simulink model "model1"  (R2024a)
settings: Solver=ode23t  StartTime=0.0  StopTime=TimeMax  MaxStep=0.1  RelTol=1e-3
model workspace (MAT data in the model file):
  con = [27 27 27 27 27 27 27 28 28 27 27 28 28 28 27 28 28 28 28 28 28 27 28 28 29 27 29 27 27 27 21 21 21 22 21 21 21 22 21 21 21 21 21 21 21 21 22 21 22 22 21 21 21 22 22 22 22 21 22 25]
  liat = [28 27 27 29 29 28 28 28 29 29 28 30 28 27 28 28 27 29 28 28 27 28 29 29 27 27 27 27 27 28 28 29 28 27 29 28 29 28 29 29 28 29 29 29 29 29 28 28 28 27 29 28 29 28 28 29 29 29 27 27 28 28 28 28 27 29 28 28 28 29 29 27 28 29 28 23 23 23 25 24 24 24 24 25 24 24 23 22 23 23 23 23 24 23 23 23 24 24 23 23 23 23 23 23 24 24 24 23 23 24 24 24 24 23 24 24 25 23 24 25 24 24 24 23 23 24 24 23 24 24 24 24 23 22 22 23 24 23 23 23 24 22 23 24 24 23 23 24 23 60]
  novar = 30
  varray = [28 29 27 30 26 28 29 27 25 30 28 29 26 27 28 25 29 30 27 28 27 29 28 30 26 27 29 28 26 27 23 24 22 25 21 23 24 22 20 25 23 24 21 22 23 20 24 25 22 21 23 24 22 25 21 22 24 25 22 15]
values from neighbouring files (symbols this model uses):
  AirDensity = 1.225    [model_variables.mat]    (also in var.m)
  AttemptData = readtable('TrackModel\410-3.csv')    [var.m]
  CD = 0.1495849    [model_variables.mat]    (also in var.m)
  CRR = 0.0015    [model_variables.mat]    (also in var.m)
  DistancetoGlide = 13301    [model_variables.mat]    (also in var.m)
  FrontArea = 0.42941    [model_variables.mat]    (also in var.m)
  FrontAxle = 510.7    [model_variables.mat]    (also in var.m)
  FrontGear = 11    [model_variables.mat]    (also in var.m)
  Gravitation = 9.80665    [model_variables.mat]    (also in var.m)
  MassWheel = 1    [model_variables.mat]    (also in var.m)
  NewData = TrackData(:, {'s', 'gradient_rad'})    [var.m]
  RadiusWheel = 0.25    [model_variables.mat]    (also in var.m)
  RearAxle = 1504.27    [model_variables.mat]    (also in var.m)
  RearGear = 142    [model_variables.mat]    (also in var.m)
  SlipAngle = 0.03    [model_variables.mat]    (also in var.m)
  SpeedData = readtable('TrackModel\KMHE3Speed.csv')    [var.m]
  TrackData = readtable('Track\Path\ePrix\mincurvfinal_ePrix_nonsmoothedgrad.csv')    [var.m]
  VehicleMass = 76    [model_variables.mat]    (also in var.m)
undefined symbols (not defined in the file or in its folder): finalatt, StateData
libraries: fl_lib x18, nesl_utility x15, sdl_lib x7, ee_lib x2, batteryecm_lib x1
(part 1 of 2)
settings Model: Creator=baiqu  LastModifiedBy=baiqu
settings SolverCC: MaxConsecutiveMinStep=5  ZeroCrossAlgorithm=Adaptive  AlgebraicLoopSolver=TrustRegion
settings DataIOCC: ReturnWorkspaceOutputs=off
settings DebuggingCC: IgnoredZcDiagnostic=none

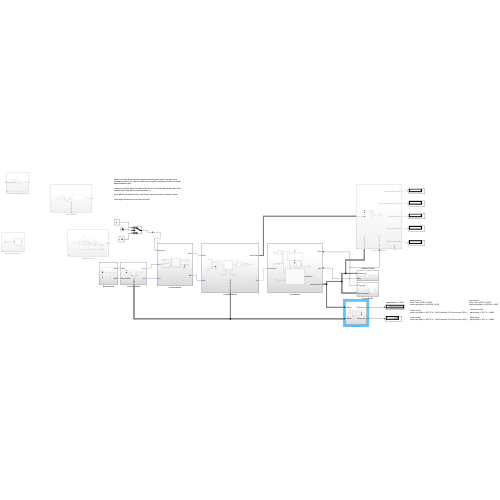
[thumbnail: Simulink's stored preview of the top-level diagram]
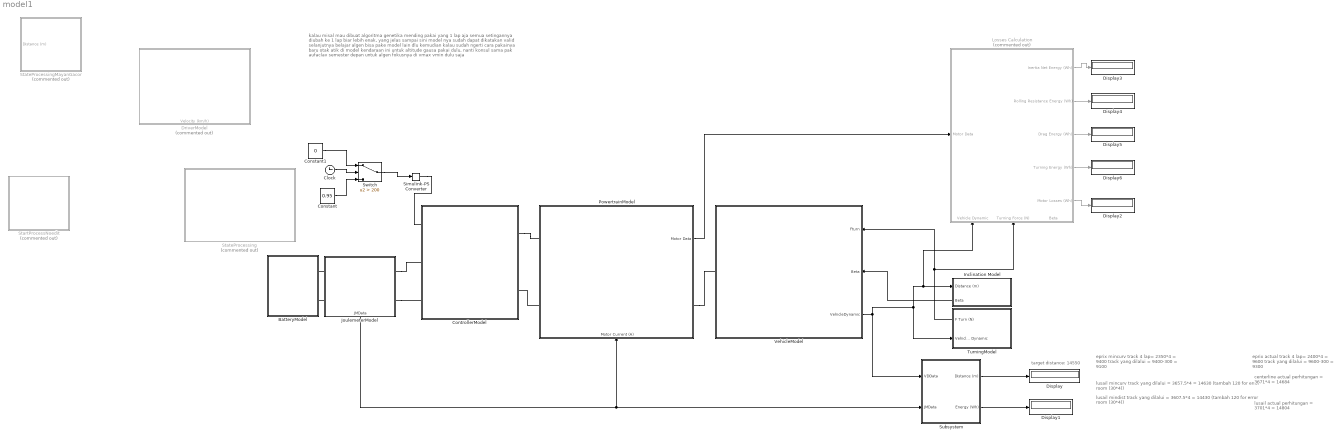
== system model1 ==
  note: target distance: 14550
  note: kalau misal mau dibuat algoritma genetika mending pakai yang 1 lap aja semua setingannya diubah ke 1 lap biar lebih enak, yang jelas sampai sini model nya sudah dapat dikatakan valid
      |
      | selanjutnya belajar algen bisa pake model lain dlu kemudian kalau sudah ngerti cara pakainya baru otak atik di model kendaraan ini
      |
      | untuk altitude gausa pakai dulu, nanti konsul sama pak aufaclav semester depan
      |
      | untuk algen fokusnya di vmax vmin dulu saja
  note: eprix actual
      | track 4 lap= 2400*4 = 9600
      | track yang dilalui = 9600-300 = 9300
  note: lusail actual
      | perhitungan = 3701*4 = 14804
  note: eprix mincurv
      | track 4 lap= 2350*4 = 9400
      | track yang dilalui = 9400-300 = 9100
  note: lusail mindist
      | track yang dilalui = 3607.5*4 = 14430 (tambah 120 for error room (30*4))
  note: lusail mincurv
      | track yang dilalui = 3657.5*4 = 14630 (tambah 120 for error room (30*4))
  note: centerline actual
      | perhitungan = 3671*4 = 14684
  BatteryModel : Subsystem
  Clock : Clock
  Constant : Constant  Value=0.95
  Constant1 : Constant  Value=0
  ControllerModel : Subsystem
  Display{,1..6} (7 alike) : Display
  DriverModel : Subsystem  Commented=on
      settings: PortSchema="{\"entries\":[{\"content\":{\"sides\":[{\"content\":{},\"type\":\"ConnectorPlacement.EquallySpacedRectSide\",\"uuid\":\"89714f29-06d9-46e2-b121-09eafd11e56c\"},{\"content\":{\"connectorIds\":[\"RConn1\"],\"side\":\"RIGHT\"},\"type\":\"ConnectorPlacement.EquallySpacedRectSide\",\"uuid\":\"45c8a396-5542-43c7-a708-f386e71eba33\"},{\"content\":{\"side\":\"TOP\"},\"type\":\"ConnectorPlacement.EquallySpacedRectSide\",\"uuid\":\"8953ccf4-c3cd-467e-b5a0-b03c7ca56c90\"},{\"content\":{\"connectorIds\":[\"In1\"],\"side\":\"BOTTOM\"},\"type\":\"ConnectorPlacement.EquallySpacedRectSide\",\"uuid\":\"ab8b1a80-a65e-491d-931c-f50f5886be3d\"}]},\"type\":\"ConnectorPlacement.EquallySpacedConnector\",\"uuid\":\"4bd302de-f506-487a-9315-f217838135a7\"}],\"packageUris\":[\"http://schema.mathworks.com/mf0/Connector/R2020b\"],\"version\":\"1.0\"}"
  Inclination Model : Subsystem
      settings: PortSchema="{\"entries\":[{\"content\":{\"sides\":[{\"content\":{},\"type\":\"ConnectorPlacement.EquallySpacedRectSide\",\"uuid\":\"136e15b9-992d-4bd3-9ecd-22bc584851ec\"},{\"content\":{\"connectorIds\":[\"In1\",\"Out1\"],\"side\":\"RIGHT\"},\"type\":\"ConnectorPlacement.EquallySpacedRectSide\",\"uuid\":\"21901198-73a1-4f2b-bd2a-55a4ec918fc9\"},{\"content\":{\"side\":\"TOP\"},\"type\":\"ConnectorPlacement.EquallySpacedRectSide\",\"uuid\":\"96b62914-b1ee-40c2-9187-7fe30b0e8d87\"}]},\"type\":\"ConnectorPlacement.EquallySpacedConnector\",\"uuid\":\"3de7d7f5-6cf3-49e2-811a-f65baadaba13\"}],\"packageUris\":[\"http://schema.mathworks.com/mf0/Connector/R2020b\"],\"version\":\"1.0\"}"
  JoulemeterModel : Subsystem
      settings: PortSchema="{\"entries\":[{\"content\":{\"sides\":[{\"content\":{\"connectorIds\":[\"LConn1\",\"LConn2\"]},\"type\":\"ConnectorPlacement.EquallySpacedRectSide\",\"uuid\":\"5b7f183a-bf7a-4999-b582-2617b2cbf3b5\"},{\"content\":{\"connectorIds\":[\"RConn1\",\"RConn2\"],\"side\":\"RIGHT\"},\"type\":\"ConnectorPlacement.EquallySpacedRectSide\",\"uuid\":\"60e6a297-a548-4f80-bd0a-fa1cc363ffaf\"},{\"content\":{\"side\":\"TOP\"},\"type\":\"ConnectorPlacement.EquallySpacedRectSide\",\"uuid\":\"7f0257a8-d3f8-4392-a80f-b293aa05a497\"},{\"content\":{\"connectorIds\":[\"Out1\"],\"side\":\"BOTTOM\"},\"type\":\"ConnectorPlacement.EquallySpacedRectSide\",\"uuid\":\"bc8eaeec-fb49-4b5e-9f30-46577002e429\"}]},\"type\":\"ConnectorPlacement.EquallySpacedConnector\",\"uuid\":\"4d471f89-f217-48cc-a8db-ea855d9b8dd6\"}],\"packageUris\":[\"http://schema.mathworks.com/mf0/Connector/R2020b\"],\"version\":\"1.0\"}"
  Losses Calculation : Subsystem  Commented=on
      settings: PortSchema="{\"entries\":[{\"content\":{\"sides\":[{\"content\":{\"connectorIds\":[\"In1\"]},\"type\":\"ConnectorPlacement.EquallySpacedRectSide\",\"uuid\":\"1b3e4d1e-49e6-427b-8c70-72d72d3276fb\"},{\"content\":{\"connectorIds\":[\"Out1\",\"Out2\",\"Out3\",\"Out4\",\"Out5\"],\"side\":\"RIGHT\"},\"type\":\"ConnectorPlacement.EquallySpacedRectSide\",\"uuid\":\"db691218-5a1c-4b6a-822c-f6125d5f80f1\"},{\"content\":{\"side\":\"TOP\"},\"type\":\"ConnectorPlacement.EquallySpacedRectSide\",\"uuid\":\"d328adc1-9cf5-4bdc-bff5-091ed8789e88\"},{\"content\":{\"connectorIds\":[\"In2\",\"In3\",\"In4\"],\"side\":\"BOTTOM\"},\"type\":\"ConnectorPlacement.EquallySpacedRectSide\",\"uuid\":\"bf96b796-aa10-4143-8481-077c36306021\"}]},\"type\":\"ConnectorPlacement.EquallySpacedConnector\",\"uuid\":\"61290827-2b1b-4af0-b2c2-32cdcb45fb74\"}],\"packageUris\":[\"http://schema.mathworks.com/mf0/Connector/R2020b\"],\"version\":\"1.0\"}"
  PowertrainModel : Subsystem
      settings: PortSchema="{\"entries\":[{\"content\":{\"sides\":[{\"content\":{\"connectorIds\":[\"LConn1\",\"LConn2\"]},\"type\":\"ConnectorPlacement.EquallySpacedRectSide\",\"uuid\":\"d69fc031-75de-46f6-9385-72f54b88d1cb\"},{\"content\":{\"connectorIds\":[\"Out1\",\"RConn1\"],\"side\":\"RIGHT\"},\"type\":\"ConnectorPlacement.EquallySpacedRectSide\",\"uuid\":\"3d253726-be1e-4202-97ec-580b8e540a5a\"},{\"content\":{\"side\":\"TOP\"},\"type\":\"ConnectorPlacement.EquallySpacedRectSide\",\"uuid\":\"cefbe44c-5e87-4e34-a220-1e2cd8a2aa2e\"},{\"content\":{\"connectorIds\":[\"In1\"],\"side\":\"BOTTOM\"},\"type\":\"ConnectorPlacement.EquallySpacedRectSide\",\"uuid\":\"e2aebd15-c630-4215-8d14-672c4b032223\"}]},\"type\":\"ConnectorPlacement.EquallySpacedConnector\",\"uuid\":\"d11a7537-5ed0-42cc-8f47-41e0a2228910\"}],\"packageUris\":[\"http://schema.mathworks.com/mf0/Connector/R2020b\"],\"version\":\"1.0\"}"
  Simulink-PS Converter : nesl_utility/Simulink-PS Converter  PhysicalDomain=network_engine_domain  SubClassName=ps_input  LeftPortType=input  RightPortType=output  PseudoPeriodic=off  Frequencies=[]  NoiseDistribution=none  NoiseParameters=[]  Unit=1  AffineConversion=off  FilteringAndDerivatives=provide  SimscapeFilterOrder=1  InputFilterTimeConstant=0.001  UdotUserProvided=0
  StartProcessNoedit : Subsystem  Commented=on
  StateProcessing : Subsystem  Commented=on
  StateProcessingMayanGacor : Subsystem  Commented=on
  Subsystem : Subsystem
  Switch : Switch  Criteria=u2 > Threshold  Threshold=200  SaturateOnIntegerOverflow=off  InputSameDT=off
  TurningModel : Subsystem
      settings: PortSchema="{\"entries\":[{\"content\":{\"sides\":[{\"content\":{\"connectorIds\":[\"Out1\",\"In1\"]},\"type\":\"ConnectorPlacement.EquallySpacedRectSide\",\"uuid\":\"d4692372-87e9-4ce8-a189-eb5e05ef7ce2\"},{\"content\":{\"side\":\"RIGHT\"},\"type\":\"ConnectorPlacement.EquallySpacedRectSide\",\"uuid\":\"c6a7fc47-7281-4ca2-ad0e-ceadd6b2be83\"},{\"content\":{\"side\":\"TOP\"},\"type\":\"ConnectorPlacement.EquallySpacedRectSide\",\"uuid\":\"b8ded78c-a4e7-43a6-a6ec-269e22706b6e\"}]},\"type\":\"ConnectorPlacement.EquallySpacedConnector\",\"uuid\":\"a77bfcc2-1edf-497f-8c86-74b621a681e7\"}],\"packageUris\":[\"http://schema.mathworks.com/mf0/Connector/R2020b\"],\"version\":\"1.0\"}"
  VehicleModel : Subsystem
      settings: PortSchema="{\"entries\":[{\"content\":{\"sides\":[{\"content\":{\"connectorIds\":[\"LConn1\"]},\"type\":\"ConnectorPlacement.EquallySpacedRectSide\",\"uuid\":\"93bb66e9-fe50-4a31-bb73-2398351c668b\"},{\"content\":{\"connectorIds\":[\"In1\",\"In2\",\"Out1\"],\"side\":\"RIGHT\"},\"type\":\"ConnectorPlacement.EquallySpacedRectSide\",\"uuid\":\"0cd3e741-0813-4587-beb9-127565be059b\"},{\"content\":{\"side\":\"TOP\"},\"type\":\"ConnectorPlacement.EquallySpacedRectSide\",\"uuid\":\"8c668a08-9049-4798-9275-4c55ebdb510f\"}]},\"type\":\"ConnectorPlacement.EquallySpacedConnector\",\"uuid\":\"e7ef1dcb-e51f-4722-9d73-8e83c911e490\"}],\"packageUris\":[\"http://schema.mathworks.com/mf0/Connector/R2020b\"],\"version\":\"1.0\"}"
  wires:
  JoulemeterModel/1(JMData) -> PowertrainModel/1(Motor Current (A)), Subsystem/2(JMData)
  TurningModel/1(F Turn (N)) -> VehicleModel/1(Fturn), Losses Calculation/3(Turning Force (N))
  Subsystem/1(Distance (m)) -> Display/1
  Subsystem/2(Energy (Wh)) -> Display1/1
  VehicleModel/1(VehicleDynamic) -> Losses Calculation/2(Vehicle Dynamic), Inclination Model/1(Distance (m)), TurningModel/1(Vehicle Dynamic), Subsystem/1(VDData)
  PowertrainModel/1(Motor Data) -> Losses Calculation/1(Motor Data)
  Losses Calculation/4(Turning Energy (Wh)) -> Display6/1
  Losses Calculation/3(Drag Energy (Wh)) -> Display5/1
  Losses Calculation/2(Rolling Resistance Energy (Wh)) -> Display4/1
  Losses Calculation/1(Inertia Net Energy (Wh)) -> Display3/1
  Inclination Model/1(Beta) -> VehicleModel/2(Beta)
  Losses Calculation/5(Motor Losses (Wh)) -> Display2/1
  Switch/1 -> Simulink-PS Converter/1
  Clock/1 -> Switch/2
  Constant1/1 -> Switch/1
  Constant/1 -> Switch/3
  connections:
  PowertrainModel/LConn2 -- ControllerModel/RConn2
  ControllerModel/RConn1 -- PowertrainModel/LConn1
  PowertrainModel/RConn1 -- VehicleModel/LConn1
  JoulemeterModel/RConn1 -- ControllerModel/LConn2
  JoulemeterModel/RConn2 -- ControllerModel/LConn3
  JoulemeterModel/LConn1 -- BatteryModel/RConn1
  JoulemeterModel/LConn2 -- BatteryModel/RConn2
  Simulink-PS Converter/RConn1 -- ControllerModel/LConn1

== system model1/BatteryModel ==
  Battery : batteryecm_lib/Battery  Vnom=Vnom V  prm_dir=simscape.enum.battery.prm_dir.disabled  R1_dis=2 Ohm  R1_ch=2 Ohm  R1=RintBat mOhm  prm_AH=simscape.enum.battery.prm_AH.infinite  AH=50 A*hr  V1=11.5 V  AH1=25 A*hr  prm_R2=simscape.enum.battery.prm_R2.disabled  R2=2000 Ohm  Tmeas=298.15 K  charge_measurement_port=simscape.enum.battery.enable.no  prm_dyn=simscape.enum.battery.prm_dyn.off  Rp1=0.005 Ohm  tau1=30 s  Rp2=0.005 Ohm  tau2=30 s  Rp3=0.005 Ohm  tau3=30 s  Rp4=0.005 Ohm  tau4=30 s  Rp5=0.005 Ohm  tau5=30 s  prm_fade=simscape.enum.battery.prm_fade.disabled  N_fade=100  AH_fade=45 A*hr  R1_fade=2.02 Ohm  R1_ch_fade=2.02 Ohm  V1_fade=10.35 V  prm_age=simscape.enum.battery.prm_age.disabled  prm_age_OCV=simscape.enum.battery.prm_age_OCV.OCV  OCV_age=0.9  SOC_age=60  Tmeas_age=298.15 K  delta_time_age_vec=[0] d  temperature_age_vec=[273] K  OCV_scaling_age=2.2134e6  OCV_offset_age=1.632e6  temp_exp_age=0.515833569 V  t_exp_age=0.75  Vnom_T2=12 V  R1_T2=2.2 Ohm  R1_T2_dis=2.2 Ohm  R1_T2_ch=2.2 Ohm  V1_T2=11.4 V  R2_T2=2200 Ohm  Rp1_T2=0.005 Ohm  tau1_T2=30 s  Rp2_T2=0.005 Ohm  tau2_T2=30 s  Rp3_T2=0.005 Ohm  tau3_T2=30 s  Rp4_T2=0.005 Ohm  tau4_T2=30 s  Rp5_T2=0.005 Ohm  tau5_T2=30 s  Tmeas2=273.15 K  thermal_port=simscape.enum.thermaleffects.omit  thermal_mass=30000 J/K  i_specify=off  i_priority=None  i=0 A  i_nominal_specify=off  i_nominal_value=1  i_nominal_unit=A  v_specify=off  v_priority=None  v=0 V  v_nominal_specify=off  v_nominal_value=1  v_nominal_unit=V  charge_specify=off  charge_priority=High  charge=50 A*hr  charge_nominal_specify=off  charge_nominal_value=1  charge_nominal_unit=A*hr  num_cycles_specify=off  num_cycles_priority=High  num_cycles=0  num_cycles_nominal_specify=off  num_cycles_nominal_value=1  num_cycles_nominal_unit=1  temperature_specify=off  temperature_priority=High  temperature=298.15 K  temperature_nominal_specify=off  temperature_nominal_value=1  temperature_nominal_unit=K
  Electrical Reference : fl_lib/Electrical/Electrical Elements/Electrical Reference
  Solver Configuration : nesl_utility/Solver Configuration  PhysicalDomain=network_engine_domain  SubClassName=solver  LeftPortType=input  RightPortType=generic  Tones=[]  Harmonics=[]  SimulateNoise=off  Profile=off  UseLocalSampling=off  EnableSwitchedLinearOptims=on  FrequencyDomain=off  UseCCode=off  RelTol=0.001  AbsTol=0.001  MinStep=1e-09  ToWorkspace=off  RevertToSquareIcSolve=off  NumHomotopyIterations=100  PhasorMode=off  PhasorModeNumHarmonics=1  ConsistencySolver=NEWTON_XTOL_AFTER_FTOL  IndexReductionMethod=DerivativeReplacement  DoDC=off  ResidualTolerance=1e-09  ConsistencyTolSource=GLOBAL  ConsistencyAbsTol=0.001  ConsistencyRelTol=0.001  ConsistencyTolFactor=0.001  UseLocalSolver=off  LocalSolverChoice=NE_BACKWARD_EULER_ADVANCER  ResolveIndetEquations=on  FunctionEvalNumThread=1  LocalSolverSampleTime=0.001  DoFixedCost=off  MaxNonlinIter=3  MaxModeIter=2  ComputeImpulses=off  ImpulseIterations=2  LinearAlgebra=auto  LinearAlgebraNumThread=0  EquationFormulation=NE_TIME_EF  DelaysMemoryBudget=1024  AutomaticFiltering=on  FilteringTimeConstant=0.001  PartitionStorageMethod=AS_NEEDED  PartitionMemoryBudget=1024  PartitionMethod=ROBUST  MultibodyUseLocalSolver=off  MultibodyLocalSolverChoice=ODE1  MultibodyLocalSolverSampleTime=0.001
  Vbus : PMIOPort  Side=Right
  GND : PMIOPort  Port=2  Side=Right
  connections:
  Battery/RConn1 -- GND/RConn1 -- Solver Configuration/RConn1 -- Electrical Reference/LConn1
  Vbus/RConn1 -- Battery/LConn1

== system model1/ControllerModel ==
  Average-Value DC-DC Converter : ee_lib/Semiconductors & Converters/Converters/Average-Value DC-DC Converter  control_option=ee.enum.converters.controlinput.dutycycle  converter_type=ee.enum.converters.dcdctype.buck  efficiency_option=ee.enum.converters.efficiency.constant  efficiency_fixed=100  i_vec=[0, 2, 5] A  efficiency_vec=[90, 95, 98]
      settings: InternalSimscapePortConfiguration="{\"Bottom\":[],\"Left\":[{\"id\":\"DutyCycle\",\"label\":\"DutyCycle\",\"type\":\"input\"},{\"id\":\"p1\",\"label\":\"1+\",\"type\":\"foundation.electrical.electrical\"},{\"id\":\"n1\",\"label\":\"1-\",\"type\":\"foundation.electrical.electrical\"}],\"Right\":[{\"id\":\"p2\",\"label\":\"2+\",\"type\":\"foundation.electrical.electrical\"},{\"id\":\"n2\",\"label\":\"2-\",\"type\":\"foundation.electrical.electrical\"}],\"Top\":[]}"
  Electrical Reference : fl_lib/Electrical/Electrical Elements/Electrical Reference
  DutyCycle : PMIOPort  Side=Left
  Con+ : PMIOPort  Port=2  Side=Left
  Con- : PMIOPort  Port=3  Side=Left
  Mot+ : PMIOPort  Port=4  Side=Right
  Mot- : PMIOPort  Port=5  Side=Right
  connections:
  Average-Value DC-DC Converter/RConn1 -- Mot+/RConn1
  Average-Value DC-DC Converter/LConn1 -- DutyCycle/RConn1
  Average-Value DC-DC Converter/LConn2 -- Con+/RConn1
  Average-Value DC-DC Converter/RConn2 -- Electrical Reference/LConn1 -- Mot-/RConn1
  Average-Value DC-DC Converter/LConn3 -- Con-/RConn1

== system model1/DriverModel ==
  Velocity (km/h) : Inport
  Bus Selector : BusSelector  OutputSignals=Velocity (km/h)
  Constant : Constant  Value=[29 29 28 29 28 28 28 29 29 28 29 28 28 29 28 28 29 27 28 28 28 28 28 28 28 28 28 28 28 28 28 28 29 28 29 28 27 28 29 27 28 28 28 28 28 28 28 29 28 29 28 28 29 29 29 29 27 29 28 28 28 28 28 29 29 28 28 28 29 29 24 23 23 23 23 23 24 25 24 23 23 23 23 23 24 23 23 23 23 23 24 24 24 24 24 24 24 23 24 23 23 24 24 24 24 23 23 23 23 23 23 23 24 24 23 23 23 24 24 23 24 24 25 24 24 22 23 23 23 23 23 23 23 23 24 24 23 24 24 56]
  Constant1 : Constant  Value=70
  MATLAB Function : MATLAB Function  TreatAsAtomicUnit=on
  Memory : Memory
  Memory1 : Memory
  Subsystem : Subsystem
  Transfer Fcn : TransferFcn  Denominator=[1e-10 1]
  DC : PMIOPort  Side=Right
  wires:
  Velocity (km/h)/1 -> Bus Selector/1
  MATLAB Function/1(control) -> Subsystem/1(state)
  MATLAB Function/3(n) -> Memory/1
  Memory1/1 -> MATLAB Function/4(state_prev)
  Memory/1 -> MATLAB Function/5(n_prev)
  Constant1/1 -> MATLAB Function/1(no_var)
  Constant/1 -> MATLAB Function/2(v_array)
  MATLAB Function/2(state) -> Memory1/1
  Bus Selector/1 -> Transfer Fcn/1  "<Velocity (km/h)>"
  Transfer Fcn/1 -> MATLAB Function/3(v)
  connections:
  DC/RConn1 -- Subsystem/RConn1

== system model1/Inclination Model ==
  note: pakai 20
  Distance (m) : Inport
  1-D Lookup Table1 : Lookup_n-D  NumberOfTableDimensions=1  BreakpointsForDimension1=NewData{:,1}  Table=NewData{:,2}  InternalRulePriority=Speed  RndMeth=Simplest
  Bus Selector : BusSelector  OutputSignals=Distance (m),Velocity (km/h)
  Constant : Constant  Value=NewData{end,1}
  Gain : Gain  Gain=1/100
  MATLAB Function1 : MATLAB Function  TreatAsAtomicUnit=on
  Unit Delay : UnitDelay  SampleTime=-1  HasFrameUpgradeWarning=on
  Beta : Outport
  wires:
  MATLAB Function1/1(position) -> 1-D Lookup Table1/1
  Constant/1 -> MATLAB Function1/2(s_track)
  Distance (m)/1 -> Bus Selector/1
  Bus Selector/1 -> Unit Delay/1  "<Distance (m)>"
  1-D Lookup Table1/1 -> Gain/1
  Gain/1 -> Beta/1
  Unit Delay/1 -> MATLAB Function1/1(s)

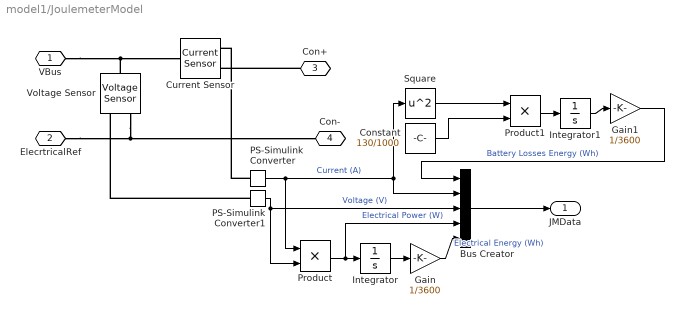
== system model1/JoulemeterModel ==
  Bus Creator : BusCreator  Inputs=5
  Constant : Constant  Value=130/1000
  Current Sensor : fl_lib/Electrical/Electrical Sensors/Current Sensor
  Gain : Gain  Gain=1/3600
  Gain1 : Gain  Gain=1/3600
  Integrator : Integrator
  Integrator1 : Integrator
  PS-Simulink Converter : nesl_utility/PS-Simulink Converter  PhysicalDomain=network_engine_domain  SubClassName=ps_output  LeftPortType=input  RightPortType=output  PseudoPeriodic=off  Frequencies=[]  VectorFormat=1-D array  Unit=A  AffineConversion=off
  PS-Simulink Converter1 : nesl_utility/PS-Simulink Converter  PhysicalDomain=network_engine_domain  SubClassName=ps_output  LeftPortType=input  RightPortType=output  PseudoPeriodic=off  Frequencies=[]  VectorFormat=1-D array  Unit=V  AffineConversion=off
  Product : Product
  Product1 : Product
  Square : Math  Operator=square
  Voltage Sensor : fl_lib/Electrical/Electrical Sensors/Voltage Sensor
  VBus : PMIOPort  Side=Left
  ElecrtricalRef : PMIOPort  Port=2  Side=Left
  Con+ : PMIOPort  Port=3  Side=Right
  Con- : PMIOPort  Port=4  Side=Right
  JMData : Outport
  wires:
  PS-Simulink Converter/1 -> Product/1, Square/1, Bus Creator/2  "Current (A)"
  PS-Simulink Converter1/1 -> Product/2, Bus Creator/3  "Voltage (V)"
  Bus Creator/1 -> JMData/1
  Product/1 -> Integrator/1, Bus Creator/4  "Electrical Power (W)"
  Gain/1 -> Bus Creator/5  "Electrical Energy (Wh)"
  Integrator/1 -> Gain/1
  Constant/1 -> Product1/2
  Square/1 -> Product1/1
  Gain1/1 -> Bus Creator/1  "Battery Losses Energy (Wh)"
  Integrator1/1 -> Gain1/1
  Product1/1 -> Integrator1/1
  connections:
  Voltage Sensor/LConn1 -- VBus/RConn1 -- Current Sensor/LConn1
  Voltage Sensor/RConn2 -- ElecrtricalRef/RConn1 -- Con-/RConn1
  PS-Simulink Converter1/LConn1 -- Voltage Sensor/RConn1
  PS-Simulink Converter/LConn1 -- Current Sensor/RConn1
  Con+/RConn1 -- Current Sensor/RConn2

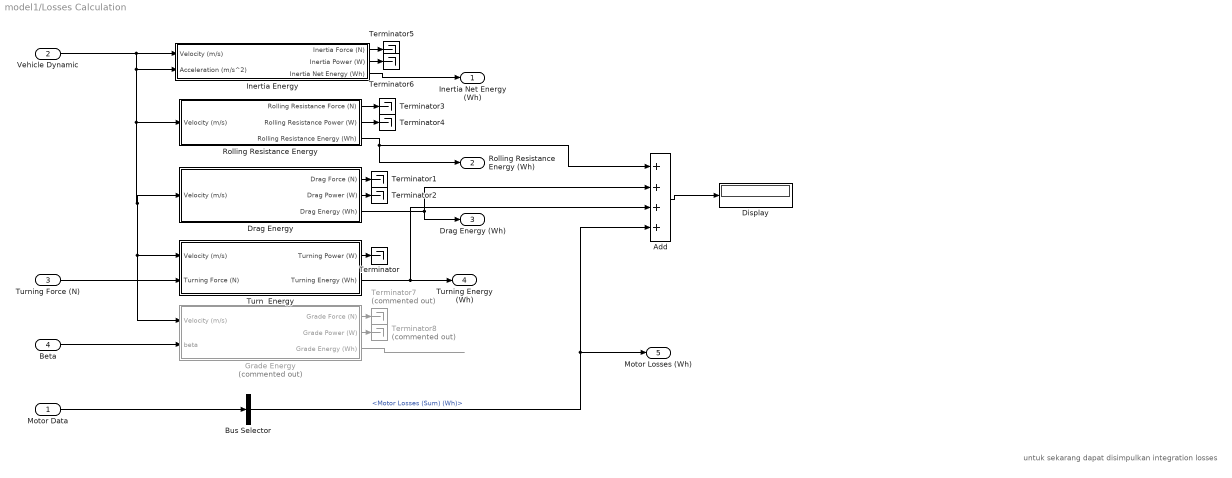
== system model1/Losses Calculation ==
  note: untuk sekarang dapat disimpulkan integration losses
  Motor Data : Inport
  Vehicle Dynamic : Inport  Port=2
  Turning Force (N) : Inport  Port=3
  Beta : Inport  Port=4
  Add : Sum  Inputs=++++
  Bus Selector : BusSelector  OutputSignals=Motor Losses (Sum) (Wh)
  Display : Display
  Drag Energy : Subsystem
  Grade Energy : Subsystem  Commented=on
  Inertia Energy : Subsystem
  Rolling Resistance Energy : Subsystem
  Terminator{,1..6} (7 alike) : Terminator
  Terminator7 : Terminator  Commented=on
  Terminator8 : Terminator  Commented=on
  Turn  Energy : Subsystem
  Inertia Net Energy (Wh) : Outport
  Rolling Resistance Energy (Wh) : Outport  Port=2
  Drag Energy (Wh) : Outport  Port=3
  Turning Energy (Wh) : Outport  Port=4
  Motor Losses (Wh) : Outport  Port=5
  wires:
  Drag Energy/2(Drag Power (W)) -> Terminator2/1
  Inertia Energy/2(Inertia Power (W)) -> Terminator6/1
  Turn  Energy/1(Turning Power (W)) -> Terminator/1
  Inertia Energy/3(Inertia Net Energy (Wh)) -> Inertia Net Energy (Wh)/1
  Drag Energy/1(Drag Force (N)) -> Terminator1/1
  Rolling Resistance Energy/3(Rolling Resistance Energy (Wh)) -> Rolling Resistance Energy (Wh)/1, Add/1
  Vehicle Dynamic/1 -> Grade Energy/1(Velocity (m/s)), Turn  Energy/1(Velocity (m/s)), Drag Energy/1(Velocity (m/s)), Rolling Resistance Energy/1(Velocity (m/s)), Inertia Energy/2(Acceleration (m/s^2)), Inertia Energy/1(Velocity (m/s))
  Rolling Resistance Energy/1(Rolling Resistance Force (N)) -> Terminator3/1
  Inertia Energy/1(Inertia Force (N)) -> Terminator5/1
  Rolling Resistance Energy/2(Rolling Resistance Power (W)) -> Terminator4/1
  Drag Energy/3(Drag Energy (Wh)) -> Drag Energy (Wh)/1, Add/2
  Turn  Energy/2(Turning Energy (Wh)) -> Add/3, Turning Energy (Wh)/1
  Add/1 -> Display/1
  Motor Data/1 -> Bus Selector/1
  Bus Selector/1 -> Add/4, Motor Losses (Wh)/1  "<Motor Losses (Sum) (Wh)>"
  Turning Force (N)/1 -> Turn  Energy/2(Turning Force (N))
  Beta/1 -> Grade Energy/2(beta)
  Grade Energy/3(Grade Energy (Wh)) -> ?
  Grade Energy/1(Grade Force (N)) -> Terminator7/1
  Grade Energy/2(Grade Power (W)) -> Terminator8/1

== system model1/PowertrainModel ==
  Motor Current (A) : Inport
  DC Motor : ee_lib/Electromechanical/Brushed Motors/DC Motor  Tag={'toolbox/physmod/elec/library/m/ee_lib_parts';'Electromechanical/Brushed_Motors/DC_Motor/Maxon/RE_65_388987_48.xml'}  field_option=ee.enum.field_option.pm  Rf=100 % Parameter not set Ohm  Lf=1 % Parameter not set H  Laf=0.15 % Parameter not set H  If0=0 % Parameter not set A  parameterization=ee.enum.dcparam_option.circuit_param  Ra=0.365 Ohm  La=0.161 mH  emf_or_torque=ee.enum.emf_or_torque.ki  Kv=12.88053 % Parameter estimated mV/rpm  Ki=123 mN*m/A  T_stall=0.24e-3 % Parameter not set N*m  w_max=19100 % Parameter not set rpm  w_rated=15000 % Parameter not set rpm  P_rated=0.08 % Parameter not set W  V_rated=1.5 % Parameter not set V  lam_param=ee.enum.lam_param.current  i_noload=0.289 A  V_i_noload=48 V  J=1340 g*cm^2  lam=0 % % Parameter not set mN*m/(rad/s)  speed0=0 % Parameter not set rpm  enable_fault_armature=simscape.enum.onoff.off  rev_faulted=1 / 3 % Parameter not set  G_faulted_armature=1e-5 % Parameter not set S  fault_trigger_armature=ee.enum.faults.faultTrigger.temporal  t_fault_armature=1 % Parameter not set s  max_permissible_current_armature=inf % Parameter not set A  t_fail_on_current_armature=1 % Parameter not set s  enable_fault_field=simscape.enum.onoff.off  G_faulted_field=1e-5 % Parameter not set S  fault_trigger_field=ee.enum.faults.faultTrigger.temporal  t_fault_field=1 % Parameter not set s  max_permissible_current_field=inf % Parameter not set A  t_fail_on_current_field=1 % Parameter not set s  fault_action=simscape.enum.assert.action.none  alpha=3.93e-3 % Parameter not set 1/K  Tmeas=25 % Parameter not set degC  thermal_mass=667.588357588358 % Parameter estimated J/K  initial_temperature=25 % Parameter not set degC
      settings: AttributesFormatString=Maxon:RE_65_388987_48
  Mechanical Rotational Reference : fl_lib/Mechanical/Rotational Elements/Mechanical Rotational Reference
  Simple Gear : sdl_lib/Gears/Simple Gear  ratio=RearGear/FrontGear  rotation_direction=sdl.enum.shaftOutputDirection.same  enable_faults=simscape.enum.onoff.off  efficiency_fault=0.05  fault_angles=pi / 12 rad  friction_model=sdl.enum.gear_efficiencies_load.off  T_noload=0.1 N*m  T_nom=5 N*m  efficiency_nom=0.8  efficiency=1  temperature_TLU=[280, 300, 320] K  load_TLU=[1, 5, 10] N*m  efficiency_TLU=[.95, .9, .85]  efficiency_TLU2=[.85, .8, .75; .95, .9, .85; .85, .8, .7]  w_thr=0.01 rad/s  pwr_thr=0.001 W  enable_backlash=false  hardstop_model=simscape.enum.hardstop.smooth  backlash_distance=1e-3 mm  r_base=0.1 m  transition=1e-4 mm  backlash_stiffness=1e6 N/m  backlash_damping=1e3 N*s/m  coeff_rest=0.7  v_tol=0.001 m/s  f_tol=0.001 N  mu_visc=[0, 0] N*m*s/rad  thermal_mass=50 J/K  temperature_specify=off  temperature_priority=High  temperature=300 K  temperature_nominal_specify=off  temperature_nominal_value=1  temperature_nominal_unit=K  x_backlash_specify=off  x_backlash_priority=None  x_backlash=0 mm  x_backlash_nominal_specify=off  x_backlash_nominal_value=1  x_backlash_nominal_unit=mm  f_hardstop_specify=off  f_hardstop_priority=None  f_hardstop=0 N  f_hardstop_nominal_specify=off  f_hardstop_nominal_value=1  f_hardstop_nominal_unit=N  v_backlash_specify=off  v_backlash_priority=None  v_backlash=0 m/s  v_backlash_nominal_specify=off  v_backlash_nominal_value=1  v_backlash_nominal_unit=m/s
  Subsystem : Subsystem
      settings: PortSchema="{\"entries\":[{\"content\":{\"sides\":[{\"content\":{\"connectorIds\":[\"LConn1\"]},\"type\":\"ConnectorPlacement.EquallySpacedRectSide\",\"uuid\":\"463aa60b-2f6b-4e46-abba-6391ca900fc1\"},{\"content\":{\"connectorIds\":[\"RConn1\"],\"side\":\"RIGHT\"},\"type\":\"ConnectorPlacement.EquallySpacedRectSide\",\"uuid\":\"74810462-e2fe-4474-8d12-7da7488b37b7\"},{\"content\":{\"side\":\"TOP\"},\"type\":\"ConnectorPlacement.EquallySpacedRectSide\",\"uuid\":\"9ca63a10-37fe-40e8-90a6-6ffb710daa85\"},{\"content\":{\"connectorIds\":[\"In1\",\"Out1\"],\"side\":\"BOTTOM\"},\"type\":\"ConnectorPlacement.EquallySpacedRectSide\",\"uuid\":\"4a0dfd4d-c60c-4da6-9cb2-0c75fefe531d\"}]},\"type\":\"ConnectorPlacement.EquallySpacedConnector\",\"uuid\":\"9b7b66d7-db13-410e-bbb4-25d259d45c14\"}],\"packageUris\":[\"http://schema.mathworks.com/mf0/Connector/R2020b\"],\"version\":\"1.0\"}"
  Unidirectional Clutch : sdl_lib/Clutches/Unidirectional Clutch  transmission_direction=sdl.enum.hubRingDirection.positive  initial_state_locked=sdl.enum.initial_lock.unlocked
      settings: InternalSimscapePortConfiguration="{\"Bottom\":[],\"Left\":[{\"id\":\"H\",\"label\":\"H\",\"type\":\"foundation.mechanical.rotational.rotational\"}],\"Right\":[{\"id\":\"R\",\"label\":\"R\",\"type\":\"foundation.mechanical.rotational.rotational\"}],\"Top\":[]}"
  Mot+ : PMIOPort  Side=Left
  Mot- : PMIOPort  Port=2  Side=Left
  Tire : PMIOPort  Port=3  Side=Right
  Motor Data : Outport
  wires:
  Motor Current (A)/1 -> Subsystem/1(Motor Current (A))
  Subsystem/1(Motor Data) -> Motor Data/1
  connections:
  Mechanical Rotational Reference/LConn1 -- DC Motor/RConn2
  DC Motor/RConn1 -- Mot-/RConn1
  DC Motor/LConn1 -- Mot+/RConn1
  Unidirectional Clutch/LConn1 -- Simple Gear/RConn1
  Unidirectional Clutch/RConn1 -- Tire/RConn1
  Subsystem/RConn1 -- Simple Gear/LConn1
  DC Motor/LConn2 -- Subsystem/LConn1

== system model1/StartProcessNoedit ==
  1-D Lookup Table : Lookup_n-D  NumberOfTableDimensions=1  BreakpointsForDimension1=StateData{1:1988,1}  IndexSearchMethod=Linear search  Table=StateData{1:1988,6}  InterpMethod=Flat  InternalRulePriority=Speed  RndMeth=Simplest
  Clock1 : Clock
  wires:
  Clock1/1 -> 1-D Lookup Table/1

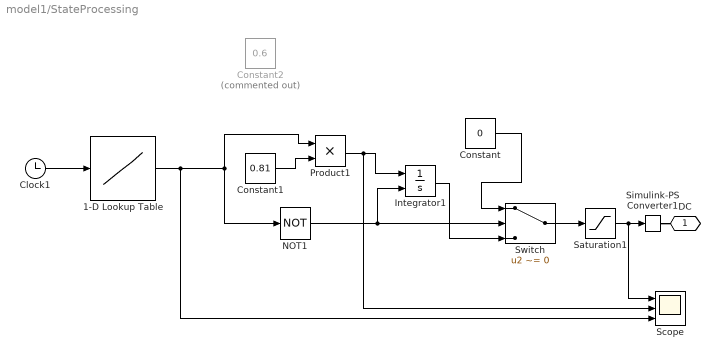
== system model1/StateProcessing ==
  1-D Lookup Table : Lookup_n-D  NumberOfTableDimensions=1  BreakpointsForDimension1=AttemptData{:,1}  IndexSearchMethod=Linear search  Table=AttemptData{:,6}  InterpMethod=Flat  InternalRulePriority=Speed  RndMeth=Simplest
  Clock1 : Clock
  Constant : Constant  Value=0
  Constant1 : Constant  Value=0.81
  Constant2 : Constant  Commented=on  Value=0.6
  Integrator1 : Integrator  ExternalReset=rising
  NOT1 : Logic  Operator=NOT  IconShape=distinctive  AllPortsSameDT=off  OutDataTypeStr=boolean
  Product1 : Product
  Saturation1 : Saturate  UpperLimit=0.95  LowerLimit=0
  Scope : Scope  NumInputPorts=3
  Simulink-PS Converter1 : nesl_utility/Simulink-PS Converter  PhysicalDomain=network_engine_domain  SubClassName=ps_input  LeftPortType=input  RightPortType=output  PseudoPeriodic=off  Frequencies=[]  NoiseDistribution=none  NoiseParameters=[]  Unit=1  AffineConversion=off  FilteringAndDerivatives=provide  SimscapeFilterOrder=1  InputFilterTimeConstant=0.001  UdotUserProvided=0
  Switch : Switch  Criteria=u2 ~= 0  SaturateOnIntegerOverflow=off  InputSameDT=off
  DC : PMIOPort  Side=Right
  wires:
  Clock1/1 -> 1-D Lookup Table/1
  Saturation1/1 -> Scope/1, Simulink-PS Converter1/1
  1-D Lookup Table/1 -> Scope/3, Product1/1, NOT1/1
  Product1/1 -> Scope/2, Integrator1/1
  NOT1/1 -> Switch/2, Integrator1/2
  Integrator1/1 -> Switch/3
  Constant/1 -> Switch/1
  Switch/1 -> Saturation1/1
  Constant1/1 -> Product1/2
  connections:
  Simulink-PS Converter1/RConn1 -- DC/RConn1

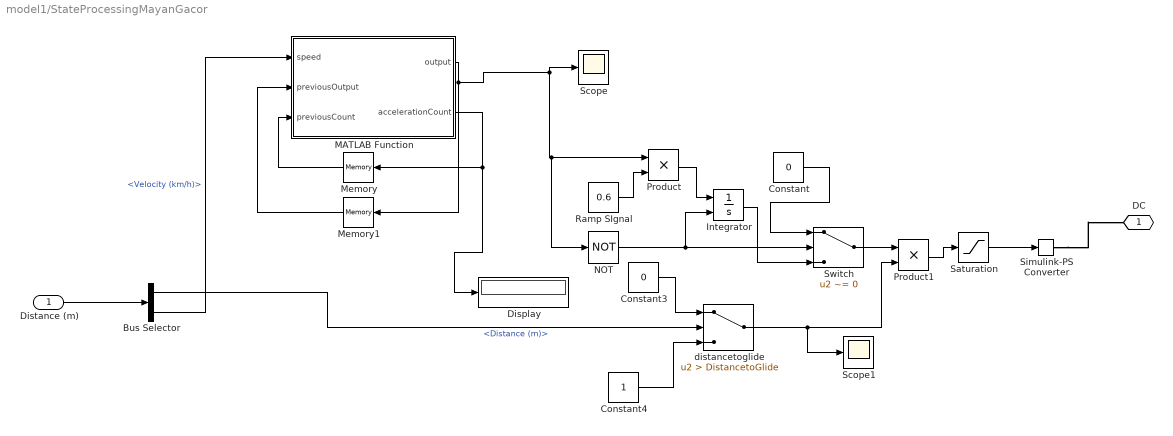
== system model1/StateProcessingMayanGacor ==
  Distance (m) : Inport
  Bus Selector : BusSelector  OutputSignals=Distance (m),Velocity (km/h)
  Constant : Constant  Value=0
  Constant3 : Constant  Value=0
  Constant4 : Constant
  Display : Display
  Integrator : Integrator  ExternalReset=rising
  MATLAB Function : MATLAB Function  TreatAsAtomicUnit=on
  Memory : Memory
  Memory1 : Memory
  NOT : Logic  Operator=NOT  IconShape=distinctive  AllPortsSameDT=off  OutDataTypeStr=boolean
  Product : Product
  Product1 : Product
  Ramp SIgnal : Constant  Value=0.6
  Saturation : Saturate  UpperLimit=0.95  LowerLimit=0
  Scope : Scope
  Scope1 : Scope
  Simulink-PS Converter : nesl_utility/Simulink-PS Converter  PhysicalDomain=network_engine_domain  SubClassName=ps_input  LeftPortType=input  RightPortType=output  PseudoPeriodic=off  Frequencies=[]  NoiseDistribution=none  NoiseParameters=[]  Unit=1  AffineConversion=off  FilteringAndDerivatives=provide  SimscapeFilterOrder=1  InputFilterTimeConstant=0.001  UdotUserProvided=0
  Switch : Switch  Criteria=u2 ~= 0  SaturateOnIntegerOverflow=off  InputSameDT=off
  distancetoglide : Switch  Criteria=u2 > Threshold  Threshold=DistancetoGlide  SaturateOnIntegerOverflow=off  InputSameDT=off
  DC : PMIOPort  Side=Right
  wires:
  Switch/1 -> Product1/1
  Ramp SIgnal/1 -> Product/2
  Saturation/1 -> Simulink-PS Converter/1
  Product/1 -> Integrator/1
  NOT/1 -> Switch/2, Integrator/2
  Constant/1 -> Switch/1
  Integrator/1 -> Switch/3
  Bus Selector/1 -> distancetoglide/2  "<Distance (m)>"
  Distance (m)/1 -> Bus Selector/1
  Constant3/1 -> distancetoglide/1
  Constant4/1 -> distancetoglide/3
  distancetoglide/1 -> Scope1/1, Product1/2
  Product1/1 -> Saturation/1
  Bus Selector/2 -> MATLAB Function/1(speed)  "<Velocity (km/h)>"
  MATLAB Function/1(output) -> Memory1/1, NOT/1, Product/1, Scope/1
  Memory1/1 -> MATLAB Function/2(previousOutput)
  MATLAB Function/2(accelerationCount) -> Memory/1, Display/1
  Memory/1 -> MATLAB Function/3(previousCount)
  connections:
  Simulink-PS Converter/RConn1 -- DC/RConn1

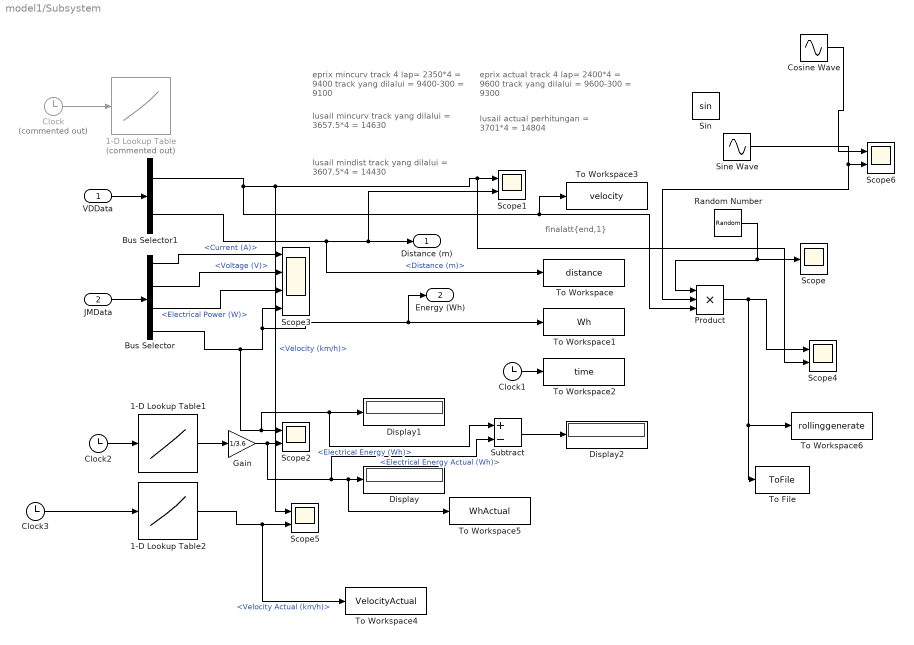
== system model1/Subsystem ==
  note: finalatt{end,1}
  note: eprix mincurv
      | track 4 lap= 2350*4 = 9400
      | track yang dilalui = 9400-300 = 9100
  note: eprix actual
      | track 4 lap= 2400*4 = 9600
      | track yang dilalui = 9600-300 = 9300
  note: lusail mincurv
      | track yang dilalui = 3657.5*4 = 14630
  note: lusail mindist
      | track yang dilalui = 3607.5*4 = 14430
  note: lusail actual
      | perhitungan = 3701*4 = 14804
  VDData : Inport
  JMData : Inport  Port=2
  1-D Lookup Table : Lookup_n-D  Commented=on  NumberOfTableDimensions=1  BreakpointsForDimension1=finalatt{:,1}  Table=finalatt{:,2}  InternalRulePriority=Speed  RndMeth=Simplest
  1-D Lookup Table1 : Lookup_n-D  NumberOfTableDimensions=1  BreakpointsForDimension1=AttemptData{:,1}  Table=AttemptData{:,5}  InternalRulePriority=Speed  RndMeth=Simplest
  1-D Lookup Table2 : Lookup_n-D  NumberOfTableDimensions=1  BreakpointsForDimension1=SpeedData{:,1}  Table=SpeedData{:,2}  InternalRulePriority=Speed  RndMeth=Simplest
  Bus Selector : BusSelector  OutputSignals=Current (A),Voltage (V),Electrical Power (W),Electrical Energy (Wh)
  Bus Selector1 : BusSelector  OutputSignals=Velocity (km/h),Distance (m)
  Clock : Clock  Commented=on
  Clock1 : Clock
  Clock2 : Clock
  Clock3 : Clock
  Cosine Wave : Sin  Amplitude=0.2  Bias=1  Frequency=0.03  Phase=pi/2  SampleTime=0
  Display : Display
  Display1 : Display
  Display2 : Display
  Gain : Gain  Gain=1/3.6
  Product : Product  Inputs=3
  Random Number : RandomNumber  Mean=1  Variance=0.0001  Seed=93939393  SampleTime=1
  Scope : Scope
  Scope{1..2,4..6} (5 alike) : Scope  NumInputPorts=2
  Scope3 : Scope  NumInputPorts=4
  Sin : Trigonometry
  Sine Wave : Sin  Amplitude=0.15  Bias=1  Frequency=0.03  SampleTime=0
  Subtract : Sum  Inputs=+-
  To File : ToFile  SaveFormat=Timeseries
  To Workspace : ToWorkspace  VariableName=distance  SampleTime=-1
      settings: Save2DSignal=2-D array (concatenate along first dimension)
  To Workspace1 : ToWorkspace  VariableName=Wh  SampleTime=-1
      settings: Save2DSignal=2-D array (concatenate along first dimension)
  To Workspace2 : ToWorkspace  VariableName=time  SampleTime=-1
      settings: Save2DSignal=2-D array (concatenate along first dimension)
  To Workspace3 : ToWorkspace  VariableName=velocity  SampleTime=-1
      settings: Save2DSignal=2-D array (concatenate along first dimension)
  To Workspace4 : ToWorkspace  VariableName=VelocityActual  SaveFormat=Timeseries  SampleTime=-1
  To Workspace5 : ToWorkspace  VariableName=WhActual  SaveFormat=Timeseries  SampleTime=-1
  To Workspace6 : ToWorkspace  VariableName=rollinggenerate  SaveFormat=Timeseries  SampleTime=-1
      settings: Decimation=10
  Distance (m) : Outport
  Energy (Wh) : Outport  Port=2
  wires:
  JMData/1 -> Bus Selector/1
  VDData/1 -> Bus Selector1/1
  Bus Selector1/1 -> Product/3, To Workspace3/1, Scope4/2, Scope1/1, Scope5/1  "<Velocity (km/h)>"
  Bus Selector1/2 -> To Workspace/1, Scope1/2, Distance (m)/1  "<Distance (m)>"
  Bus Selector/3 -> Scope3/3  "<Electrical Power (W)>"
  Bus Selector/2 -> Scope3/2  "<Voltage (V)>"
  Bus Selector/1 -> Scope3/1  "<Current (A)>"
  Bus Selector/4 -> Subtract/1, Display1/1, Scope2/1, Energy (Wh)/1, To Workspace1/1, Scope3/4  "<Electrical Energy (Wh)>"
  Clock/1 -> 1-D Lookup Table/1
  Clock1/1 -> To Workspace2/1
  1-D Lookup Table1/1 -> Gain/1
  Clock2/1 -> 1-D Lookup Table1/1
  Gain/1 -> Subtract/2, To Workspace5/1, Display/1, Scope2/2  "<Electrical Energy Actual (Wh)>"
  Subtract/1 -> Display2/1
  Random Number/1 -> Product/1, Scope/1
  Product/1 -> To File/1, To Workspace6/1, Scope4/1
  1-D Lookup Table2/1 -> To Workspace4/1, Scope5/2  "<Velocity Actual (km/h)>"
  Clock3/1 -> 1-D Lookup Table2/1
  Sine Wave/1 -> Product/2, Scope6/2
  Cosine Wave/1 -> Scope6/1

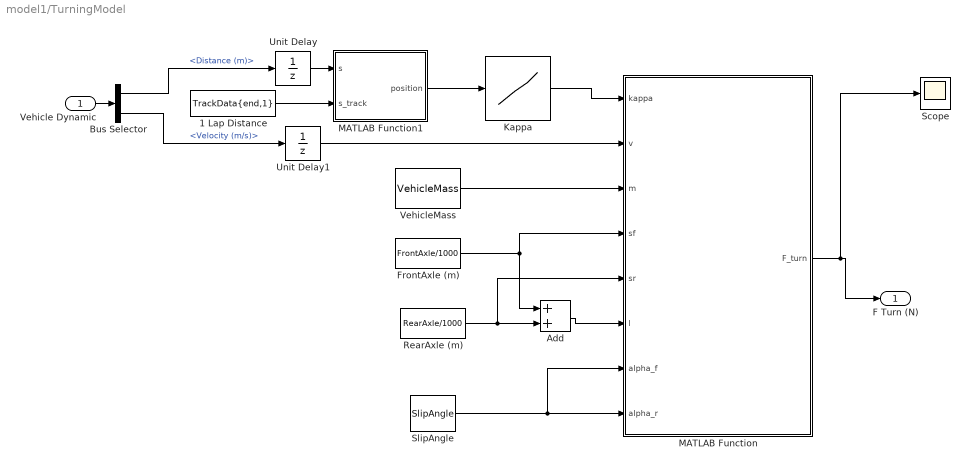
== system model1/TurningModel ==
  Vehicle Dynamic : Inport
  1 Lap Distance : Constant  Value=TrackData{end,1}
  Add : Sum
  Bus Selector : BusSelector  OutputSignals=Distance (m),Velocity (m/s)
  FrontAxle (m) : Constant  Value=FrontAxle/1000
  Kappa : Lookup_n-D  NumberOfTableDimensions=1  BreakpointsForDimension1=TrackData{:,1}  Table=TrackData{:,4}  InterpMethod=Flat  InternalRulePriority=Speed  RndMeth=Simplest
  MATLAB Function : MATLAB Function  TreatAsAtomicUnit=on
  MATLAB Function1 : MATLAB Function  TreatAsAtomicUnit=on
  RearAxle (m) : Constant  Value=RearAxle/1000
  Scope : Scope
  SlipAngle : Constant  Value=SlipAngle
  Unit Delay : UnitDelay  SampleTime=-1  HasFrameUpgradeWarning=on
  Unit Delay1 : UnitDelay  SampleTime=-1  HasFrameUpgradeWarning=on
  VehicleMass : Constant  Value=VehicleMass
  F Turn (N) : Outport
  wires:
  VehicleMass/1 -> MATLAB Function/3(m)
  1 Lap Distance/1 -> MATLAB Function1/2(s_track)
  Kappa/1 -> MATLAB Function/1(kappa)
  RearAxle (m)/1 -> MATLAB Function/5(sr), Add/2
  FrontAxle (m)/1 -> MATLAB Function/4(sf), Add/1
  Bus Selector/1 -> Unit Delay/1  "<Distance (m)>"
  MATLAB Function1/1(position) -> Kappa/1
  SlipAngle/1 -> MATLAB Function/7(alpha_f), MATLAB Function/8(alpha_r)
  MATLAB Function/1(F_turn) -> Scope/1, F Turn (N)/1
  Vehicle Dynamic/1 -> Bus Selector/1
  Bus Selector/2 -> Unit Delay1/1  "<Velocity (m/s)>"
  Add/1 -> MATLAB Function/6(l)
  Unit Delay/1 -> MATLAB Function1/1(s)
  Unit Delay1/1 -> MATLAB Function/2(v)

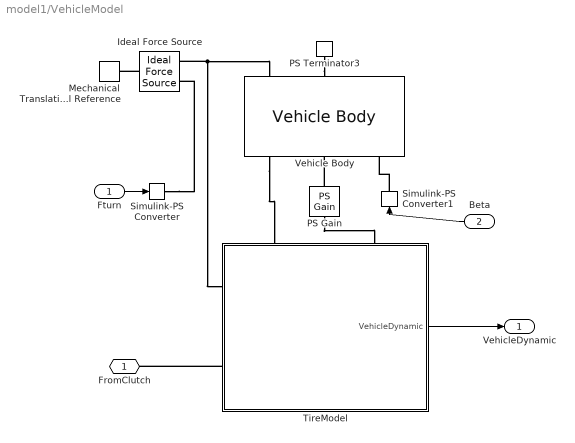
== system model1/VehicleModel ==
  Fturn : Inport
  Beta : Inport  Port=2
  Ideal Force Source : fl_lib/Mechanical/Mechanical Sources/Ideal Force Source
  Mechanical Translational Reference : fl_lib/Mechanical/Translational Elements/Mechanical Translational Reference
  PS Gain : fl_lib/Physical Signals/Functions/PS Gain  gain=0.5
  PS Terminator3 : fl_lib/Physical Signals/Sinks/PS Terminator
  Simulink-PS Converter : nesl_utility/Simulink-PS Converter  PhysicalDomain=network_engine_domain  SubClassName=ps_input  LeftPortType=input  RightPortType=output  PseudoPeriodic=off  Frequencies=[]  NoiseDistribution=none  NoiseParameters=[]  Unit=N  AffineConversion=off  FilteringAndDerivatives=provide  SimscapeFilterOrder=1  InputFilterTimeConstant=0.001  UdotUserProvided=0
  Simulink-PS Converter1 : nesl_utility/Simulink-PS Converter  PhysicalDomain=network_engine_domain  SubClassName=ps_input  LeftPortType=input  RightPortType=output  PseudoPeriodic=off  Frequencies=[]  NoiseDistribution=none  NoiseParameters=[]  Unit=rad  AffineConversion=off  FilteringAndDerivatives=provide  SimscapeFilterOrder=1  InputFilterTimeConstant=0.001  UdotUserProvided=0
  TireModel : Subsystem
      settings: PortSchema="{\"entries\":[{\"content\":{\"sides\":[{\"content\":{\"connectorIds\":[\"LConn1\",\"LConn2\"]},\"type\":\"ConnectorPlacement.EquallySpacedRectSide\",\"uuid\":\"ad88246c-79e4-4500-822e-5fea39c5896c\"},{\"content\":{\"connectorIds\":[\"Out1\"],\"side\":\"RIGHT\"},\"type\":\"ConnectorPlacement.EquallySpacedRectSide\",\"uuid\":\"913d52ca-54a5-4560-b3df-e1f57975974a\"},{\"content\":{\"connectorIds\":[\"LConn3\",\"LConn4\"],\"side\":\"TOP\"},\"type\":\"ConnectorPlacement.EquallySpacedRectSide\",\"uuid\":\"5900099e-62c2-49ce-8123-88bd27d24a29\"}]},\"type\":\"ConnectorPlacement.EquallySpacedConnector\",\"uuid\":\"881a997e-2d63-4bf2-b975-40b530568104\"}],\"packageUris\":[\"http://schema.mathworks.com/mf0/Connector/R2020b\"],\"version\":\"1.0\"}"
  Vehicle Body : sdl_lib/Tires & Vehicles/Vehicle Body  mass=VehicleMass kg  n_w=1  x_f=FrontAxle mm  x_r=RearAxle mm  y_c=GroundClearance mm  mass_var=simscape.enum.onoff.off  g=9.81 m/s^2  liftoff_warning=simscape.enum.onoff.off  area=FrontArea m^2  Cd=CD  rho=1.18 kg/m^3  model_pitch=simscape.enum.onoff.off  inertia=4000 kg*m^2  suspension_model=sdl.enum.linearTLU.linear  k_f=1e4 N/m  b_f=1e4 N*s/m  k_r=1e4 N/m  b_r=1e4 N*s/m  k_f_TLU=[-2000, -1000, 0, 1000, 2000] N  x_f_TLU=[-.4, -.2, 0, .2, .4] m  b_f_TLU=[-200, -100, 0, 100, 200] N  v_f_TLU=[-4, -2, 0, 2, 4] m/s  k_r_TLU=[-2000, -1000, 0, 1000, 2000] N  x_r_TLU=[-.4, -.2, 0, .2, .4] m  b_r_TLU=[-200, -100, 0, 100, 200] N  v_r_TLU=[-4, -2, 0, 2, 4] m/s  interp_method=simscape.enum.interpolation.linear  extrap_method=simscape.enum.extrapolation.linear  model_hardstop=simscape.enum.onoff.off  upper_bound_f=.25 m  lower_bound_f=-.25 m  stop_k_f=1e6 N/m  stop_b_f=150 N*s/m  upper_bound_r=.25 m  lower_bound_r=-.25 m  stop_k_r=1e6 N/m  stop_b_r=150 N*s/m  initial_pitch=0 rad  initial_pitch_rate=0 rad/s  v_specify=off  v_priority=High  v=0 m/s  v_nominal_specify=off  v_nominal_value=1  v_nominal_unit=m/s
  FromClutch : PMIOPort  Side=Left
  VehicleDynamic : Outport
  wires:
  TireModel/1(VehicleDynamic) -> VehicleDynamic/1
  Fturn/1 -> Simulink-PS Converter/1
  Beta/1 -> Simulink-PS Converter1/1
  connections:
  TireModel/LConn2 -- FromClutch/RConn1
  Vehicle Body/RConn1 -- TireModel/LConn3
  Ideal Force Source/LConn1 -- Mechanical Translational Reference/LConn1
  Ideal Force Source/RConn2 -- TireModel/LConn1 -- Vehicle Body/LConn1
  Simulink-PS Converter/RConn1 -- Ideal Force Source/RConn1
  PS Terminator3/LConn1 -- Vehicle Body/LConn2
  PS Gain/LConn1 -- Vehicle Body/RConn2
  PS Gain/RConn1 -- TireModel/LConn4
  Simulink-PS Converter1/RConn1 -- Vehicle Body/RConn3

== system model1/DriverModel/Subsystem ==
  state : Inport
  Constant : Constant  Value=0
  Constant1 : Constant  Value=0.6
  Integrator1 : Integrator  ExternalReset=rising
  NOT1 : Logic  Operator=NOT  IconShape=distinctive  AllPortsSameDT=off  OutDataTypeStr=boolean
  Product1 : Product
  Saturation1 : Saturate  UpperLimit=0.95  LowerLimit=0
  Scope : Scope  NumInputPorts=3
  Simulink-PS Converter1 : nesl_utility/Simulink-PS Converter  PhysicalDomain=network_engine_domain  SubClassName=ps_input  LeftPortType=input  RightPortType=output  PseudoPeriodic=off  Frequencies=[]  NoiseDistribution=none  NoiseParameters=[]  Unit=1  AffineConversion=off  FilteringAndDerivatives=provide  SimscapeFilterOrder=1  InputFilterTimeConstant=0.001  UdotUserProvided=0
  Switch : Switch  Criteria=u2 ~= 0  SaturateOnIntegerOverflow=off  InputSameDT=off
  DC : PMIOPort  Side=Right
  wires:
  Integrator1/1 -> Scope/1, Switch/3
  Switch/1 -> Saturation1/1
  NOT1/1 -> Switch/2, Integrator1/2
  Constant/1 -> Switch/1
  state/1 -> Product1/1, NOT1/1
  Saturation1/1 -> Scope/2, Simulink-PS Converter1/1
  Constant1/1 -> Product1/2
  Product1/1 -> Scope/3, Integrator1/1
  connections:
  Simulink-PS Converter1/RConn1 -- DC/RConn1

== system model1/Losses Calculation/Drag Energy ==
  Velocity (m/s) : Inport
  Bus Selector : BusSelector  OutputSignals=Velocity (m/s)
  Constant : Constant  Value=1/2*FrontArea*CD*AirDensity
  Gain : Gain  Gain=1/3600
  Integrator : Integrator
  Product : Product  Inputs=3
  Product1 : Product
  Drag Force (N) : Outport
  Drag Power (W) : Outport  Port=2
  Drag Energy (Wh) : Outport  Port=3
  wires:
  Velocity (m/s)/1 -> Bus Selector/1
  Product/1 -> Drag Force (N)/1, Product1/1  "Drag Force (N)"
  Product1/1 -> Drag Power (W)/1, Integrator/1  "Drag Power (W)"
  Constant/1 -> Product/1
  Integrator/1 -> Gain/1  "Drag Energy (J)"
  Gain/1 -> Drag Energy (Wh)/1
  Bus Selector/1 -> Product/2, Product/3, Product1/2  "<Velocity (m/s)>"

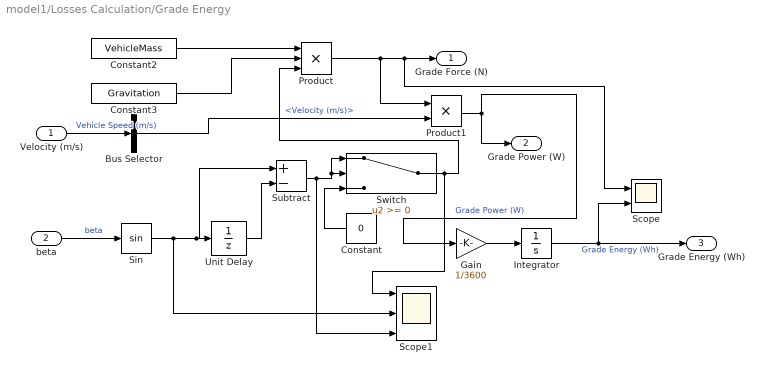
== system model1/Losses Calculation/Grade Energy ==
  Velocity (m/s) : Inport
  beta : Inport  Port=2
  Bus Selector : BusSelector  OutputSignals=Velocity (m/s)
  Constant : Constant  Value=0
  Constant2 : Constant  Value=VehicleMass
  Constant3 : Constant  Value=Gravitation
  Gain : Gain  Gain=1/3600
  Integrator : Integrator
  Product : Product  Inputs=3
  Product1 : Product
  Scope : Scope  NumInputPorts=2
  Scope1 : Scope  NumInputPorts=3
  Sin : Trigonometry
  Subtract : Sum  Inputs=+-
  Switch : Switch  SaturateOnIntegerOverflow=off  InputSameDT=off
  Unit Delay : UnitDelay  SampleTime=-1  HasFrameUpgradeWarning=on
  Grade Force (N) : Outport
  Grade Power (W) : Outport  Port=2
  Grade Energy (Wh) : Outport  Port=3
  wires:
  Gain/1 -> Integrator/1
  Velocity (m/s)/1 -> Bus Selector/1  "Vehicle Speed (m/s)"
  Constant2/1 -> Product/1
  Constant3/1 -> Product/2
  beta/1 -> Sin/1  "beta"
  Sin/1 -> Scope1/2, Subtract/1, Unit Delay/1
  Product/1 -> Product1/1, Scope/1, Grade Force (N)/1
  Bus Selector/1 -> Product1/2  "<Velocity (m/s)>"
  Product1/1 -> Gain/1, Grade Power (W)/1  "Grade Power (W)"
  Integrator/1 -> Scope/2, Grade Energy (Wh)/1  "Grade Energy (Wh)"
  Unit Delay/1 -> Subtract/2
  Subtract/1 -> Scope1/3, Switch/1, Switch/2
  Constant/1 -> Switch/3
  Switch/1 -> Scope1/1, Product/3

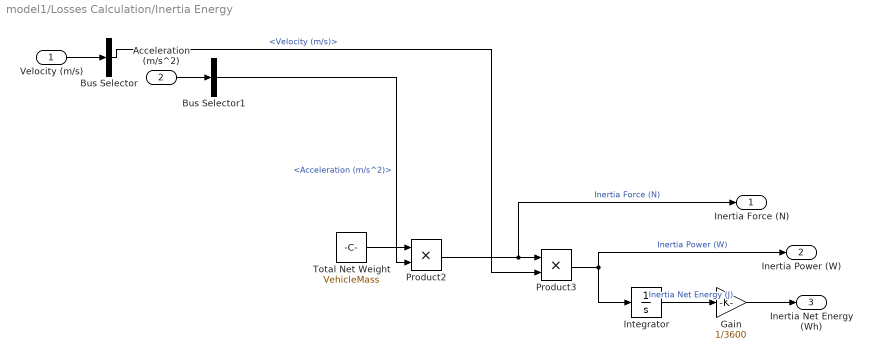
== system model1/Losses Calculation/Inertia Energy ==
  Velocity (m/s) : Inport
  Acceleration (m/s^2) : Inport  Port=2
  Bus Selector : BusSelector  OutputSignals=Velocity (m/s)
  Bus Selector1 : BusSelector  OutputSignals=Acceleration (m/s^2)
  Gain : Gain  Gain=1/3600
  Integrator : Integrator
  Product2 : Product
  Product3 : Product
  Total Net Weight : Constant  Value=VehicleMass
  Inertia Force (N) : Outport
  Inertia Power (W) : Outport  Port=2
  Inertia Net Energy (Wh) : Outport  Port=3
  wires:
  Product3/1 -> Inertia Power (W)/1, Integrator/1  "Inertia Power (W)"
  Total Net Weight/1 -> Product2/1
  Integrator/1 -> Gain/1  "Inertia Net Energy (J)"
  Acceleration (m/s^2)/1 -> Bus Selector1/1
  Product2/1 -> Inertia Force (N)/1, Product3/1  "Inertia Force (N)"
  Velocity (m/s)/1 -> Bus Selector/1
  Gain/1 -> Inertia Net Energy (Wh)/1
  Bus Selector/1 -> Product3/2  "<Velocity (m/s)>"
  Bus Selector1/1 -> Product2/2  "<Acceleration (m/s^2)>"

== system model1/Losses Calculation/Rolling Resistance Energy ==
  Velocity (m/s) : Inport
  Bus Selector : BusSelector  OutputSignals=Velocity (m/s)
  Constant2 : Constant  Value=VehicleMass
  Constant3 : Constant  Value=Gravitation
  Constant4 : Constant  Value=CRR
  Gain : Gain  Gain=1/3600
  Integrator : Integrator
  Product2 : Product
  Product3 : Product  Inputs=3
  Rolling Resistance Force (N) : Outport
  Rolling Resistance Power (W) : Outport  Port=2
  Rolling Resistance Energy (Wh) : Outport  Port=3
  wires:
  Product2/1 -> Rolling Resistance Power (W)/1, Integrator/1  "Rolling Resistance Power (W)"
  Velocity (m/s)/1 -> Bus Selector/1
  Integrator/1 -> Gain/1  "Rolling Resistance Energy (J)"
  Gain/1 -> Rolling Resistance Energy (Wh)/1
  Bus Selector/1 -> Product2/1  "<Velocity (m/s)>"
  Constant3/1 -> Product3/2
  Constant2/1 -> Product3/1
  Constant4/1 -> Product3/3
  Product3/1 -> Rolling Resistance Force (N)/1, Product2/2

== system model1/Losses Calculation/Turn  Energy ==
  Velocity (m/s) : Inport
  Turning Force (N) : Inport  Port=2
  Bus Selector : BusSelector  OutputSignals=Velocity (m/s)
  Gain : Gain  Gain=1/3600
  Integrator : Integrator
  Product1 : Product
  Turning Power (W) : Outport
  Turning Energy (Wh) : Outport  Port=2
  wires:
  Product1/1 -> Turning Power (W)/1, Integrator/1  "Turning Power (W)"
  Integrator/1 -> Gain/1  "Turning Energy (J)"
  Gain/1 -> Turning Energy (Wh)/1
  Turning Force (N)/1 -> Product1/2  "Turning Force (N)"
  Velocity (m/s)/1 -> Bus Selector/1  "Vehicle Speed (m/s)"
  Bus Selector/1 -> Product1/1  "<Velocity (m/s)>"
